simulink model "Fig520"  (R2014b)
settings: Solver=ode3  StartTime=0.0  StopTime=0.1048576  FixedStep=2e-7  RelTol=1e-3
libraries: commseqgen2 x1, commanapbnd3 x1, commrandsrc2 x1
settings Model: Creator=Silage  LastModifiedBy=Silage

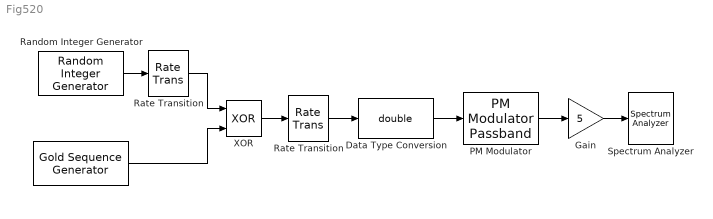
== system Fig520 ==
  " " : commseqgen2/Gold Sequence Generator  genPoly1=[1 0 0 1 0 1]  iniState1=[1 1 1 0 1]  genPoly2=[1 1 1 1 0 1]  iniState2=[1 0 0 0 1]  index=0  shift=0  outVarSiz=off  maxOutSizeMode=Dialog parameter  maxOutSize=[10 1]  ts=5e-5  frameBased=off  sampPerFrame=1  reset=off  outDataType=double
  Data Type Conversion : DataTypeConversion  OutDataTypeStr=double
  Gain : Gain  Gain=5
  PM Modulator : commanapbnd3/PM Modulator Passband  Fc=100000  Ph=pi  Kc=pi
  Random Integer Generator : commrandsrc2/Random Integer Generator  mul=2  seed=randseed  Ts=1e-3  frameBased=off  sampPerFrame=50  orient=on  outDataType=double
  "Rate Transition " : RateTransition  OutPortSampleTime=2e-7
  Rate Transition : RateTransition  OutPortSampleTime=5e-5
  Spectrum Analyzer : SpectrumAnalyzer
  XOR : Logic  Operator=XOR  IconShape=distinctive  AllPortsSameDT=off  OutDataTypeStr=boolean
  wires:
  " "/1 -> XOR/2
  Random Integer Generator/1 -> Rate Transition/1
  Rate Transition/1 -> XOR/1
  Data Type Conversion/1 -> PM Modulator/1
  XOR/1 -> "Rate Transition "/1
  "Rate Transition "/1 -> Data Type Conversion/1
  PM Modulator/1 -> Gain/1
  Gain/1 -> Spectrum Analyzer/1
